simulink model "gm_uz_pmsm_model_vnl"  (R2023b)
settings: Solver=FixedStepAuto  StartTime=0.0  StopTime=0.05  RelTol=1e-3
PreLoadFcn:
  | uz_pmsm_model_init_parameter
PostLoadFcn:
  | % Import the data from Excel for a lookup table
  | FluxMapData = readtable('C:\Users\Philipp\ultrazohm\ultrazohm_sw\ip_cores\uz_pmsm_model\FluxMapData_2023-05-26_13-07-57.csv');
  | % Row indices for lookup table
  | d_current_in_d_axis = FluxMapData(8:27,1:end);
  | % Column indices for lookup table
  | q_current_in_d_axis = FluxMapData(29:48,1:end);
  | % Output values for lookup table
  | d_Flux_d_axis = FluxMapData(50:69,1:end);
undefined symbols (not defined in the file or in its folder): ad1, ad2, ad3, ad4, ad5, ad6, aq1, aq2, aq3, aq4, aq5, aq6, d_current_d_Flux, d_current_q_Flux, entkopplung_dynamic, entkopplung_linear, entkopplung_static, Fid1_Giq1, Fid2_Giq2, Flux_d, Flux_q, friction_coefficient, inertia, Ki_Bo_d, Ki_Bo_q, Kp_Bo_d, Kp_Bo_q, L_d, L_q, Ldq, parameter_nachfuerung, polepair, praediktion_entkopplung_nonlinear, psi_pm, q_current_d_Flux, q_current_q_Flux, R_1, simulate_mechanical, simulate_nonlinear_modell, simulate_open_loop, static_friction_torque, tau_sum, ts, ts_regler
libraries: hdlmdlgenlib x16, slpidlib x6, simulink x4
(part 4 of 5)

== system gm_uz_pmsm_model_vnl/uz_pmsm_model/Product9 ==
  In1 : Inport
  In2 : Inport  Port=2
  Product9 : Product  Inputs=**  OutDataTypeStr=single  SampleTime=1e-08
  Product9_pd1 : Delay  DelayLength=6
  Out1 : Outport
  wires:
  Product9_pd1/1 -> Out1/1
  Product9/1 -> Product9_pd1/1
  In2/1 -> Product9/2
  In1/1 -> Product9/1

== system gm_uz_pmsm_model_vnl/uz_pmsm_model/Product91 ==
  In1 : Inport
  In2 : Inport  Port=2
  Product91 : Product  Inputs=**  OutDataTypeStr=single  SampleTime=1e-08
  Product91_pd1 : Delay  DelayLength=6
  Out1 : Outport
  wires:
  Product91_pd1/1 -> Out1/1
  Product91/1 -> Product91_pd1/1
  In2/1 -> Product91/2
  In1/1 -> Product91/1

== system gm_uz_pmsm_model_vnl/uz_pmsm_model/Product92 ==
  In1 : Inport
  In2 : Inport  Port=2
  Product92 : Product  Inputs=**  OutDataTypeStr=single  SampleTime=1e-08
  Product92_pd1 : Delay  DelayLength=6
  Out1 : Outport
  wires:
  Product92_pd1/1 -> Out1/1
  Product92/1 -> Product92_pd1/1
  In2/1 -> Product92/2
  In1/1 -> Product92/1

== system gm_uz_pmsm_model_vnl/uz_pmsm_model/Reciprocal1_recip ==
  In1 : Inport
  Reciprocal1_recip : Math  Operator=reciprocal  SampleTime=1e-08
  Reciprocal1_recip_pd1 : Delay  DelayLength=16
  Out1 : Outport
  wires:
  Reciprocal1_recip_pd1/1 -> Out1/1
  Reciprocal1_recip/1 -> Reciprocal1_recip_pd1/1
  In1/1 -> Reciprocal1_recip/1

== system gm_uz_pmsm_model_vnl/uz_pmsm_model/Reciprocal1_recip1 ==
  In1 : Inport
  Reciprocal1_recip1 : Math  Operator=reciprocal  SampleTime=1e-08
  Reciprocal1_recip1_pd1 : Delay  DelayLength=16
  Out1 : Outport
  wires:
  Reciprocal1_recip1_pd1/1 -> Out1/1
  Reciprocal1_recip1/1 -> Reciprocal1_recip1_pd1/1
  In1/1 -> Reciprocal1_recip1/1

== system gm_uz_pmsm_model_vnl/uz_pmsm_model/Reciprocal_recip ==
  In1 : Inport
  Reciprocal_recip : Math  Operator=reciprocal  SampleTime=1e-08
  Reciprocal_recip_pd1 : Delay  DelayLength=16
  Out1 : Outport
  wires:
  Reciprocal_recip_pd1/1 -> Out1/1
  Reciprocal_recip/1 -> Reciprocal_recip_pd1/1
  In1/1 -> Reciprocal_recip/1

== system gm_uz_pmsm_model_vnl/uz_pmsm_model/Reciprocal_recip1 ==
  In1 : Inport
  Reciprocal_recip1 : Math  Operator=reciprocal  SampleTime=1e-08
  Reciprocal_recip1_pd1 : Delay  DelayLength=16
  Out1 : Outport
  wires:
  Reciprocal_recip1_pd1/1 -> Out1/1
  Reciprocal_recip1/1 -> Reciprocal_recip1_pd1/1
  In1/1 -> Reciprocal_recip1/1

== system gm_uz_pmsm_model_vnl/uz_pmsm_model/Sign1 ==
  In1 : Inport
  Sign1 : Signum  SampleTime=1e-08
  Out1 : Outport
  wires:
  Sign1/1 -> Out1/1
  In1/1 -> Sign1/1

== system gm_uz_pmsm_model_vnl/uz_pmsm_model/Sum ==
  In1 : Inport
  In2 : Inport  Port=2
  Sum : Sum  OutDataTypeStr=single  SampleTime=1e-08
  Sum_pd1 : Delay  DelayLength=6
  Out1 : Outport
  wires:
  Sum_pd1/1 -> Out1/1
  Sum/1 -> Sum_pd1/1
  In2/1 -> Sum/2
  In1/1 -> Sum/1

== system gm_uz_pmsm_model_vnl/uz_pmsm_model/Sum1 ==
  In1 : Inport
  In2 : Inport  Port=2
  Sum1 : Sum  Inputs=+-  OutDataTypeStr=single  SampleTime=1e-08
  Sum1_pd1 : Delay  DelayLength=6
  Out1 : Outport
  wires:
  Sum1_pd1/1 -> Out1/1
  Sum1/1 -> Sum1_pd1/1
  In2/1 -> Sum1/2
  In1/1 -> Sum1/1

== system gm_uz_pmsm_model_vnl/uz_pmsm_model/Sum10 ==
  In1 : Inport
  In2 : Inport  Port=2
  Sum10 : Sum  Inputs=+-  OutDataTypeStr=single  SampleTime=1e-08
  Sum10_pd1 : Delay  DelayLength=6
  Out1 : Outport
  wires:
  Sum10_pd1/1 -> Out1/1
  Sum10/1 -> Sum10_pd1/1
  In2/1 -> Sum10/2
  In1/1 -> Sum10/1

== system gm_uz_pmsm_model_vnl/uz_pmsm_model/Sum101 ==
  In1 : Inport
  In2 : Inport  Port=2
  Sum101 : Sum  Inputs=+-  OutDataTypeStr=single  SampleTime=1e-08
  Sum101_pd1 : Delay  DelayLength=6
  Out1 : Outport
  wires:
  Sum101_pd1/1 -> Out1/1
  Sum101/1 -> Sum101_pd1/1
  In2/1 -> Sum101/2
  In1/1 -> Sum101/1

== system gm_uz_pmsm_model_vnl/uz_pmsm_model/Sum11 ==
  In1 : Inport
  In2 : Inport  Port=2
  Sum11 : Sum  Inputs=+-  OutDataTypeStr=single  SampleTime=1e-08
  Sum11_pd1 : Delay  DelayLength=6
  Out1 : Outport
  wires:
  Sum11_pd1/1 -> Out1/1
  Sum11/1 -> Sum11_pd1/1
  In2/1 -> Sum11/2
  In1/1 -> Sum11/1

== system gm_uz_pmsm_model_vnl/uz_pmsm_model/Sum12 ==
  In1 : Inport
  In2 : Inport  Port=2
  Sum12 : Sum  OutDataTypeStr=single  SampleTime=1e-08
  Sum12_pd1 : Delay  DelayLength=6
  Out1 : Outport
  wires:
  Sum12_pd1/1 -> Out1/1
  Sum12/1 -> Sum12_pd1/1
  In2/1 -> Sum12/2
  In1/1 -> Sum12/1

== system gm_uz_pmsm_model_vnl/uz_pmsm_model/Sum13 ==
  In1 : Inport
  In2 : Inport  Port=2
  Sum13 : Sum  OutDataTypeStr=single  SampleTime=1e-08
  Sum13_pd1 : Delay  DelayLength=6
  Out1 : Outport
  wires:
  Sum13_pd1/1 -> Out1/1
  Sum13/1 -> Sum13_pd1/1
  In2/1 -> Sum13/2
  In1/1 -> Sum13/1

== system gm_uz_pmsm_model_vnl/uz_pmsm_model/Sum14 ==
  In1 : Inport
  In2 : Inport  Port=2
  Sum14 : Sum  Inputs=+-  OutDataTypeStr=single  SampleTime=1e-08
  Sum14_pd1 : Delay  DelayLength=6
  Out1 : Outport
  wires:
  Sum14_pd1/1 -> Out1/1
  Sum14/1 -> Sum14_pd1/1
  In2/1 -> Sum14/2
  In1/1 -> Sum14/1

== system gm_uz_pmsm_model_vnl/uz_pmsm_model/Sum2 ==
  In1 : Inport
  In2 : Inport  Port=2
  Sum2 : Sum  Inputs=+-  OutDataTypeStr=single  SampleTime=1e-08
  Sum2_pd1 : Delay  DelayLength=6
  Out1 : Outport
  wires:
  Sum2_pd1/1 -> Out1/1
  Sum2/1 -> Sum2_pd1/1
  In2/1 -> Sum2/2
  In1/1 -> Sum2/1

== system gm_uz_pmsm_model_vnl/uz_pmsm_model/Sum21 ==
  In1 : Inport
  In2 : Inport  Port=2
  Sum21 : Sum  Inputs=+-  OutDataTypeStr=single  SampleTime=1e-08
  Sum21_pd1 : Delay  DelayLength=6
  Out1 : Outport
  wires:
  Sum21_pd1/1 -> Out1/1
  Sum21/1 -> Sum21_pd1/1
  In2/1 -> Sum21/2
  In1/1 -> Sum21/1

== system gm_uz_pmsm_model_vnl/uz_pmsm_model/Sum22 ==
  In1 : Inport
  In2 : Inport  Port=2
  Sum22 : Sum  Inputs=+-  OutDataTypeStr=single  SampleTime=1e-08
  Sum22_pd1 : Delay  DelayLength=6
  Out1 : Outport
  wires:
  Sum22_pd1/1 -> Out1/1
  Sum22/1 -> Sum22_pd1/1
  In2/1 -> Sum22/2
  In1/1 -> Sum22/1

== system gm_uz_pmsm_model_vnl/uz_pmsm_model/Sum23 ==
  In1 : Inport
  In2 : Inport  Port=2
  Sum23 : Sum  Inputs=+-  OutDataTypeStr=single  SampleTime=1e-08
  Sum23_pd1 : Delay  DelayLength=6
  Out1 : Outport
  wires:
  Sum23_pd1/1 -> Out1/1
  Sum23/1 -> Sum23_pd1/1
  In2/1 -> Sum23/2
  In1/1 -> Sum23/1

== system gm_uz_pmsm_model_vnl/uz_pmsm_model/Sum24 ==
  In1 : Inport
  In2 : Inport  Port=2
  Sum24 : Sum  Inputs=+-  OutDataTypeStr=single  SampleTime=1e-08
  Sum24_pd1 : Delay  DelayLength=6
  Out1 : Outport
  wires:
  Sum24_pd1/1 -> Out1/1
  Sum24/1 -> Sum24_pd1/1
  In2/1 -> Sum24/2
  In1/1 -> Sum24/1

== system gm_uz_pmsm_model_vnl/uz_pmsm_model/Sum3 ==
  In1 : Inport
  In2 : Inport  Port=2
  Sum3 : Sum  Inputs=+-  OutDataTypeStr=single  SampleTime=1e-08
  Sum3_pd1 : Delay  DelayLength=6
  Out1 : Outport
  wires:
  Sum3_pd1/1 -> Out1/1
  Sum3/1 -> Sum3_pd1/1
  In2/1 -> Sum3/2
  In1/1 -> Sum3/1

== system gm_uz_pmsm_model_vnl/uz_pmsm_model/Sum31 ==
  In1 : Inport
  In2 : Inport  Port=2
  Sum31 : Sum  Inputs=+-  OutDataTypeStr=single  SampleTime=1e-08
  Sum31_pd1 : Delay  DelayLength=6
  Out1 : Outport
  wires:
  Sum31_pd1/1 -> Out1/1
  Sum31/1 -> Sum31_pd1/1
  In2/1 -> Sum31/2
  In1/1 -> Sum31/1

== system gm_uz_pmsm_model_vnl/uz_pmsm_model/Sum32 ==
  In1 : Inport
  In2 : Inport  Port=2
  Sum32 : Sum  OutDataTypeStr=single  SampleTime=1e-08
  Sum32_pd1 : Delay  DelayLength=6
  Out1 : Outport
  wires:
  Sum32_pd1/1 -> Out1/1
  Sum32/1 -> Sum32_pd1/1
  In2/1 -> Sum32/2
  In1/1 -> Sum32/1

== system gm_uz_pmsm_model_vnl/uz_pmsm_model/Sum33 ==
  In1 : Inport
  In2 : Inport  Port=2
  Sum33 : Sum  Inputs=+-  OutDataTypeStr=single  SampleTime=1e-08
  Sum33_pd1 : Delay  DelayLength=6
  Out1 : Outport
  wires:
  Sum33_pd1/1 -> Out1/1
  Sum33/1 -> Sum33_pd1/1
  In2/1 -> Sum33/2
  In1/1 -> Sum33/1

== system gm_uz_pmsm_model_vnl/uz_pmsm_model/Sum3_stage2 ==
  In1 : Inport
  In2 : Inport  Port=2
  Sum3_stage2 : Sum  OutDataTypeStr=single  SampleTime=1e-08
  Sum3_stage2_pd1 : Delay  DelayLength=6
  Out1 : Outport
  wires:
  Sum3_stage2_pd1/1 -> Out1/1
  Sum3_stage2/1 -> Sum3_stage2_pd1/1
  In2/1 -> Sum3_stage2/2
  In1/1 -> Sum3_stage2/1

== system gm_uz_pmsm_model_vnl/uz_pmsm_model/Sum3_stage21 ==
  In1 : Inport
  In2 : Inport  Port=2
  Sum3_stage21 : Sum  Inputs=+-  OutDataTypeStr=single  SampleTime=1e-08
  Sum3_stage21_pd1 : Delay  DelayLength=6
  Out1 : Outport
  wires:
  Sum3_stage21_pd1/1 -> Out1/1
  Sum3_stage21/1 -> Sum3_stage21_pd1/1
  In2/1 -> Sum3_stage21/2
  In1/1 -> Sum3_stage21/1

== system gm_uz_pmsm_model_vnl/uz_pmsm_model/Sum3_stage3 ==
  In1 : Inport
  In2 : Inport  Port=2
  Sum3_stage3 : Sum  Inputs=+-  OutDataTypeStr=single  SampleTime=1e-08
  Sum3_stage3_pd1 : Delay  DelayLength=6
  Out1 : Outport
  wires:
  Sum3_stage3_pd1/1 -> Out1/1
  Sum3_stage3/1 -> Sum3_stage3_pd1/1
  In2/1 -> Sum3_stage3/2
  In1/1 -> Sum3_stage3/1

== system gm_uz_pmsm_model_vnl/uz_pmsm_model/Sum3_stage31 ==
  In1 : Inport
  In2 : Inport  Port=2
  Sum3_stage31 : Sum  OutDataTypeStr=single  SampleTime=1e-08
  Sum3_stage31_pd1 : Delay  DelayLength=6
  Out1 : Outport
  wires:
  Sum3_stage31_pd1/1 -> Out1/1
  Sum3_stage31/1 -> Sum3_stage31_pd1/1
  In2/1 -> Sum3_stage31/2
  In1/1 -> Sum3_stage31/1

== system gm_uz_pmsm_model_vnl/uz_pmsm_model/Sum4 ==
  In1 : Inport
  In2 : Inport  Port=2
  Sum4 : Sum  OutDataTypeStr=single  SampleTime=1e-08
  Sum4_pd1 : Delay  DelayLength=6
  Out1 : Outport
  wires:
  Sum4_pd1/1 -> Out1/1
  Sum4/1 -> Sum4_pd1/1
  In2/1 -> Sum4/2
  In1/1 -> Sum4/1

== system gm_uz_pmsm_model_vnl/uz_pmsm_model/Sum41 ==
  In1 : Inport
  In2 : Inport  Port=2
  Sum41 : Sum  OutDataTypeStr=single  SampleTime=1e-08
  Sum41_pd1 : Delay  DelayLength=6
  Out1 : Outport
  wires:
  Sum41_pd1/1 -> Out1/1
  Sum41/1 -> Sum41_pd1/1
  In2/1 -> Sum41/2
  In1/1 -> Sum41/1

== system gm_uz_pmsm_model_vnl/uz_pmsm_model/Sum4_stage2 ==
  In1 : Inport
  In2 : Inport  Port=2
  Sum4_stage2 : Sum  Inputs=+-  OutDataTypeStr=single  SampleTime=1e-08
  Sum4_stage2_pd1 : Delay  DelayLength=6
  Out1 : Outport
  wires:
  Sum4_stage2_pd1/1 -> Out1/1
  Sum4_stage2/1 -> Sum4_stage2_pd1/1
  In2/1 -> Sum4_stage2/2
  In1/1 -> Sum4_stage2/1

== system gm_uz_pmsm_model_vnl/uz_pmsm_model/Sum4_stage3 ==
  In1 : Inport
  In2 : Inport  Port=2
  Sum4_stage3 : Sum  Inputs=+-  OutDataTypeStr=single  SampleTime=1e-08
  Sum4_stage3_pd1 : Delay  DelayLength=6
  Out1 : Outport
  wires:
  Sum4_stage3_pd1/1 -> Out1/1
  Sum4_stage3/1 -> Sum4_stage3_pd1/1
  In2/1 -> Sum4_stage3/2
  In1/1 -> Sum4_stage3/1

== system gm_uz_pmsm_model_vnl/uz_pmsm_model/Sum5 ==
  In1 : Inport
  In2 : Inport  Port=2
  Sum5 : Sum  OutDataTypeStr=single  SampleTime=1e-08
  Sum5_pd1 : Delay  DelayLength=6
  Out1 : Outport
  wires:
  Sum5_pd1/1 -> Out1/1
  Sum5/1 -> Sum5_pd1/1
  In2/1 -> Sum5/2
  In1/1 -> Sum5/1

== system gm_uz_pmsm_model_vnl/uz_pmsm_model/Sum51 ==
  In1 : Inport
  In2 : Inport  Port=2
  Sum51 : Sum  Inputs=+-  OutDataTypeStr=single  SampleTime=1e-08
  Sum51_pd1 : Delay  DelayLength=6
  Out1 : Outport
  wires:
  Sum51_pd1/1 -> Out1/1
  Sum51/1 -> Sum51_pd1/1
  In2/1 -> Sum51/2
  In1/1 -> Sum51/1

== system gm_uz_pmsm_model_vnl/uz_pmsm_model/Sum52 ==
  In1 : Inport
  In2 : Inport  Port=2
  Sum52 : Sum  OutDataTypeStr=single  SampleTime=1e-08
  Sum52_pd1 : Delay  DelayLength=6
  Out1 : Outport
  wires:
  Sum52_pd1/1 -> Out1/1
  Sum52/1 -> Sum52_pd1/1
  In2/1 -> Sum52/2
  In1/1 -> Sum52/1

== system gm_uz_pmsm_model_vnl/uz_pmsm_model/Sum53 ==
  In1 : Inport
  In2 : Inport  Port=2
  Sum53 : Sum  OutDataTypeStr=single  SampleTime=1e-08
  Sum53_pd1 : Delay  DelayLength=6
  Out1 : Outport
  wires:
  Sum53_pd1/1 -> Out1/1
  Sum53/1 -> Sum53_pd1/1
  In2/1 -> Sum53/2
  In1/1 -> Sum53/1

== system gm_uz_pmsm_model_vnl/uz_pmsm_model/Sum6 ==
  In1 : Inport
  In2 : Inport  Port=2
  Sum6 : Sum  Inputs=+-  OutDataTypeStr=single  SampleTime=1e-08
  Sum6_pd1 : Delay  DelayLength=6
  Out1 : Outport
  wires:
  Sum6_pd1/1 -> Out1/1
  Sum6/1 -> Sum6_pd1/1
  In2/1 -> Sum6/2
  In1/1 -> Sum6/1

== system gm_uz_pmsm_model_vnl/uz_pmsm_model/Sum7 ==
  In1 : Inport
  In2 : Inport  Port=2
  Sum7 : Sum  Inputs=+-  OutDataTypeStr=single  SampleTime=1e-08
  Sum7_pd1 : Delay  DelayLength=6
  Out1 : Outport
  wires:
  Sum7_pd1/1 -> Out1/1
  Sum7/1 -> Sum7_pd1/1
  In2/1 -> Sum7/2
  In1/1 -> Sum7/1

== system gm_uz_pmsm_model_vnl/uz_pmsm_model/Sum71 ==
  In1 : Inport
  In2 : Inport  Port=2
  Sum71 : Sum  Inputs=+-  OutDataTypeStr=single  SampleTime=1e-08
  Sum71_pd1 : Delay  DelayLength=6
  Out1 : Outport
  wires:
  Sum71_pd1/1 -> Out1/1
  Sum71/1 -> Sum71_pd1/1
  In2/1 -> Sum71/2
  In1/1 -> Sum71/1

== system gm_uz_pmsm_model_vnl/uz_pmsm_model/Sum8 ==
  In1 : Inport
  In2 : Inport  Port=2
  Sum8 : Sum  Inputs=+-  OutDataTypeStr=single  SampleTime=1e-08
  Sum8_pd1 : Delay  DelayLength=6
  Out1 : Outport
  wires:
  Sum8_pd1/1 -> Out1/1
  Sum8/1 -> Sum8_pd1/1
  In2/1 -> Sum8/2
  In1/1 -> Sum8/1

== system gm_uz_pmsm_model_vnl/uz_pmsm_model/Tanh ==
  In1 : Inport
  Tanh : Trigonometry  Operator=tanh  SampleTime=1e-08
  Tanh_pd1 : Delay  DelayLength=25
  Out1 : Outport
  wires:
  Tanh_pd1/1 -> Out1/1
  Tanh/1 -> Tanh_pd1/1
  In1/1 -> Tanh/1

== system gm_uz_pmsm_model_vnl/uz_pmsm_model/Tanh1 ==
  In1 : Inport
  Tanh1 : Trigonometry  Operator=tanh  SampleTime=1e-08
  Tanh1_pd1 : Delay  DelayLength=25
  Out1 : Outport
  wires:
  Tanh1_pd1/1 -> Out1/1
  Tanh1/1 -> Tanh1_pd1/1
  In1/1 -> Tanh1/1

== system gm_uz_pmsm_model_vnl/uz_pmsm_model/Tanh11 ==
  In1 : Inport
  Tanh11 : Trigonometry  Operator=cosh  SampleTime=1e-08
  Tanh11_pd1 : Delay  DelayLength=17
  Out1 : Outport
  wires:
  Tanh11_pd1/1 -> Out1/1
  Tanh11/1 -> Tanh11_pd1/1
  In1/1 -> Tanh11/1

== system gm_uz_pmsm_model_vnl/uz_pmsm_model/Tanh12 ==
  In1 : Inport
  Tanh12 : Trigonometry  Operator=tanh  SampleTime=1e-08
  Tanh12_pd1 : Delay  DelayLength=25
  Out1 : Outport
  wires:
  Tanh12_pd1/1 -> Out1/1
  Tanh12/1 -> Tanh12_pd1/1
  In1/1 -> Tanh12/1

== system gm_uz_pmsm_model_vnl/uz_pmsm_model/Tanh13 ==
  In1 : Inport
  Tanh13 : Trigonometry  Operator=cosh  SampleTime=1e-08
  Tanh13_pd1 : Delay  DelayLength=17
  Out1 : Outport
  wires:
  Tanh13_pd1/1 -> Out1/1
  Tanh13/1 -> Tanh13_pd1/1
  In1/1 -> Tanh13/1

== system gm_uz_pmsm_model_vnl/uz_pmsm_model/Tanh2 ==
  In1 : Inport
  Tanh2 : Trigonometry  Operator=cosh  SampleTime=1e-08
  Tanh2_pd1 : Delay  DelayLength=17
  Out1 : Outport
  wires:
  Tanh2_pd1/1 -> Out1/1
  Tanh2/1 -> Tanh2_pd1/1
  In1/1 -> Tanh2/1

== system gm_uz_pmsm_model_vnl/uz_pmsm_model/Tanh21 ==
  In1 : Inport
  Tanh21 : Trigonometry  Operator=cosh  SampleTime=1e-08
  Tanh21_pd1 : Delay  DelayLength=17
  Out1 : Outport
  wires:
  Tanh21_pd1/1 -> Out1/1
  Tanh21/1 -> Tanh21_pd1/1
  In1/1 -> Tanh21/1

== system gm_uz_pmsm_model_vnl/uz_pmsm_model/Tanh3 ==
  In1 : Inport
  Tanh3 : Trigonometry  Operator=cosh  SampleTime=1e-08
  Tanh3_pd1 : Delay  DelayLength=17
  Out1 : Outport
  wires:
  Tanh3_pd1/1 -> Out1/1
  Tanh3/1 -> Tanh3_pd1/1
  In1/1 -> Tanh3/1

== system gm_uz_pmsm_model_vnl/uz_pmsm_model/Tanh31 ==
  In1 : Inport
  Tanh31 : Trigonometry  Operator=cosh  SampleTime=1e-08
  Tanh31_pd1 : Delay  DelayLength=17
  Out1 : Outport
  wires:
  Tanh31_pd1/1 -> Out1/1
  Tanh31/1 -> Tanh31_pd1/1
  In1/1 -> Tanh31/1

== system gm_uz_pmsm_model_vnl/uz_pmsm_model/Tanh4 ==
  In1 : Inport
  Tanh4 : Trigonometry  Operator=cosh  SampleTime=1e-08
  Tanh4_pd1 : Delay  DelayLength=17
  Out1 : Outport
  wires:
  Tanh4_pd1/1 -> Out1/1
  Tanh4/1 -> Tanh4_pd1/1
  In1/1 -> Tanh4/1

== system gm_uz_pmsm_model_vnl/uz_pmsm_model/Tanh41 ==
  In1 : Inport
  Tanh41 : Trigonometry  Operator=cosh  SampleTime=1e-08
  Tanh41_pd1 : Delay  DelayLength=17
  Out1 : Outport
  wires:
  Tanh41_pd1/1 -> Out1/1
  Tanh41/1 -> Tanh41_pd1/1
  In1/1 -> Tanh41/1

== system gm_uz_pmsm_model_vnl/uz_pmsm_model/Tanh5 ==
  In1 : Inport
  Tanh5 : Trigonometry  Operator=tanh  SampleTime=1e-08
  Tanh5_pd1 : Delay  DelayLength=25
  Out1 : Outport
  wires:
  Tanh5_pd1/1 -> Out1/1
  Tanh5/1 -> Tanh5_pd1/1
  In1/1 -> Tanh5/1

== system gm_uz_pmsm_model_vnl/uz_pmsm_model/abs ==
  In1 : Inport
  abs : Abs  SampleTime=1e-08  OutDataTypeStr=single  SaturateOnIntegerOverflow=off
  Out1 : Outport
  wires:
  abs/1 -> Out1/1
  In1/1 -> abs/1

== system gm_uz_pmsm_model_vnl/uz_pmsm_model/abs1 ==
  In1 : Inport
  abs1 : Abs  SampleTime=1e-08  OutDataTypeStr=single  SaturateOnIntegerOverflow=off
  Out1 : Outport
  wires:
  abs1/1 -> Out1/1
  In1/1 -> abs1/1

== system gm_uz_pmsm_model_vnl/uz_pmsm_model/abs2 ==
  In1 : Inport
  abs2 : Abs  SampleTime=1e-08  OutDataTypeStr=single  SaturateOnIntegerOverflow=off
  Out1 : Outport
  wires:
  abs2/1 -> Out1/1
  In1/1 -> abs2/1

== system gm_uz_pmsm_model_vnl/uz_pmsm_model/abs3 ==
  In1 : Inport
  abs3 : Abs  SampleTime=1e-08  OutDataTypeStr=single  SaturateOnIntegerOverflow=off
  Out1 : Outport
  wires:
  abs3/1 -> Out1/1
  In1/1 -> abs3/1

== system gm_uz_pmsm_model_vnl/uz_pmsm_model/abs4 ==
  In1 : Inport
  abs4 : Abs  SampleTime=1e-08  OutDataTypeStr=single  SaturateOnIntegerOverflow=off
  Out1 : Outport
  wires:
  abs4/1 -> Out1/1
  In1/1 -> abs4/1

== system gm_uz_pmsm_model_vnl/uz_pmsm_model/abs5 ==
  In1 : Inport
  abs5 : Abs  SampleTime=1e-08  OutDataTypeStr=single  SaturateOnIntegerOverflow=off
  Out1 : Outport
  wires:
  abs5/1 -> Out1/1
  In1/1 -> abs5/1

== system gm_uz_pmsm_model_vnl/uz_pmsm_model/abs6 ==
  In1 : Inport
  abs6 : Abs  SampleTime=1e-08  OutDataTypeStr=single  SaturateOnIntegerOverflow=off
  Out1 : Outport
  wires:
  abs6/1 -> Out1/1
  In1/1 -> abs6/1

== system gm_uz_pmsm_model_vnl/uz_pmsm_model/abs7 ==
  In1 : Inport
  abs7 : Abs  SampleTime=1e-08  OutDataTypeStr=single  SaturateOnIntegerOverflow=off
  Out1 : Outport
  wires:
  abs7/1 -> Out1/1
  In1/1 -> abs7/1

== system gm_uz_pmsm_model_vnl/uz_pmsm_model/abs8 ==
  In1 : Inport
  abs8 : Abs  SampleTime=1e-08  OutDataTypeStr=single  SaturateOnIntegerOverflow=off
  Out1 : Outport
  wires:
  abs8/1 -> Out1/1
  In1/1 -> abs8/1

== system gm_uz_pmsm_model_vnl/uz_pmsm_model/abs9 ==
  In1 : Inport
  abs9 : Abs  SampleTime=1e-08  OutDataTypeStr=single  SaturateOnIntegerOverflow=off
  Out1 : Outport
  wires:
  abs9/1 -> Out1/1
  In1/1 -> abs9/1

== system gm_uz_pmsm_model_vnl/uz_pmsm_model_vnl/mechanical_system ==
  note: This delay breaks the algebraic loop between mechanical and electrical system.
      | Introduces a delay of 500ns.
  reset : Inport
  M_Mi : Inport  Port=2
  mu : Inport  Port=3
  M_n0 : Inport  Port=4
  reciprocal_J : Inport  Port=5
  load_torque : Inport  Port=6
  Abs : Abs  SaturateOnIntegerOverflow=off
  Delay : Delay  DelayLength=1
  Product11 : Product
  Product12 : Product
  Product4 : Product
  Sign1 : Signum
  Sum : Sum  Inputs=|+-
  Sum1 : Sum  Inputs=|+-
  Sum5 : Sum  Inputs=|++
  integrator1 : Subsystem
  omega_mech : Outport
  wires:
  Delay/1 -> Sum1/1
  Product4/1 -> Sum/2
  Sum/1 -> Delay/1
  load_torque/1 -> Sum1/2
  Sum1/1 -> Product11/2
  M_Mi/1 -> Sum/1
  reciprocal_J/1 -> Product11/1
  M_n0/1 -> Sum5/2
  mu/1 -> Product12/1
  Product12/1 -> Sum5/1
  reset/1 -> integrator1/1(reset)
  Abs/1 -> Product12/2
  integrator1/1(outt) -> omega_mech/1, Abs/1, Sign1/1
  Sign1/1 -> Product4/2
  Sum5/1 -> Product4/1
  Product11/1 -> integrator1/2(in)

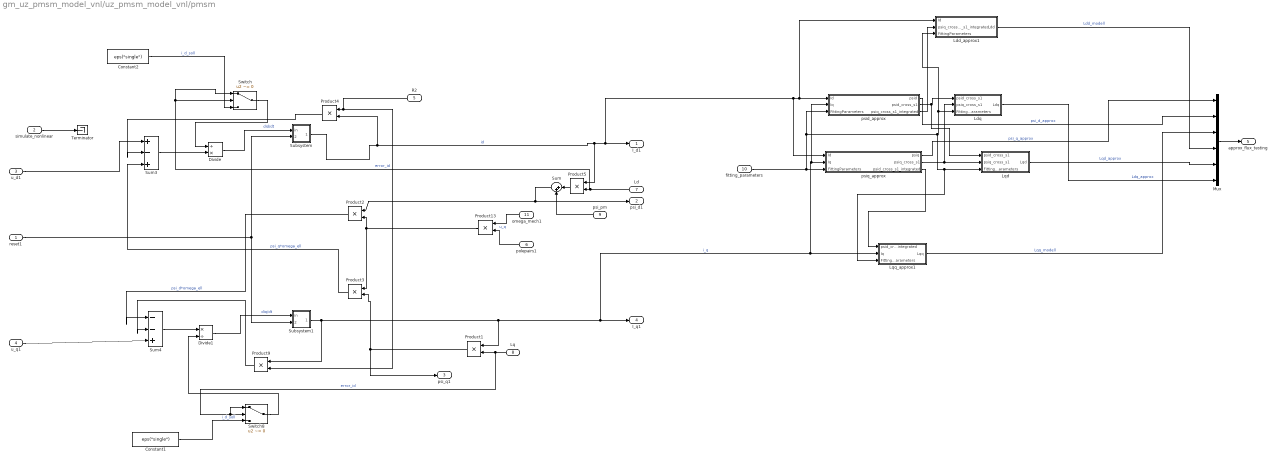
== system gm_uz_pmsm_model_vnl/uz_pmsm_model_vnl/pmsm ==
  reset1 : Inport
  simulate_nonlinear : Inport  Port=2
  u_d1 : Inport  Port=3
  u_q1 : Inport  Port=4
  R2 : Inport  Port=5
  polepairs1 : Inport  Port=6
  Ld : Inport  Port=7
  Lq : Inport  Port=8
  psi_pm : Inport  Port=9
  fitting_parameters : Inport  Port=10
  omega_mech1 : Inport  Port=11
  Constant1 : Constant  Value="eps(\"single\")"  OutDataTypeStr=single  SampleTime=ts
  Constant2 : Constant  Value="eps(\"single\")"  OutDataTypeStr=single  SampleTime=ts
  Divide : Product  Inputs=/*  OutDataTypeStr=Inherit: Same as first input
  Divide1 : Product  Inputs=*/  OutDataTypeStr=Inherit: Same as first input
  Ldd_approx1 : Subsystem
  Ldq : Subsystem
  Lqd : Subsystem
  Lqq_approx1 : Subsystem
  Mux : Mux  Inputs=6
  Product1 : Product
  Product{2,4..5,9,13} (5 alike) : Product  OutDataTypeStr=Inherit: Same as first input
  Product3 : Product
  Subsystem : Subsystem
  Subsystem1 : Subsystem
  Sum : Sum  Inputs=|++  OutDataTypeStr=Inherit: Same as first input
  Sum3 : Sum  Inputs=|+-+  OutDataTypeStr=Inherit: Same as first input
  Sum4 : Sum  Inputs=|--+
  Switch : Switch  Criteria=u2 ~= 0  Threshold="eps(\"single\")"  SaturateOnIntegerOverflow=off  InputSameDT=off
  Switch8 : Switch  Criteria=u2 ~= 0  SaturateOnIntegerOverflow=off  InputSameDT=off
  Terminator : Terminator
  psid_approx : Subsystem
  psiq_approx : Subsystem
  I_d1 : Outport
  psi_d1 : Outport  Port=2
  psi_q1 : Outport  Port=3
  I_q1 : Outport  Port=4
  approx_flux_testing : Outport  Port=5
  wires:
  fitting_parameters/1 -> psiq_approx/3(FittingParameters), psid_approx/3(FittingParameters), Ldq/3(FittingParameters), Ldd_approx1/3(FittingParameters), Lqd/3(FittingParameters), Lqq_approx1/3(FittingParameters)
  Mux/1 -> approx_flux_testing/1
  Ldd_approx1/1(Ldd) -> Mux/4  "Ldd_modell"
  psiq_approx/3(psid_cross_s1_integrated) -> Lqq_approx1/1(psid_cross_s1_integrated)
  psid_approx/3(psiq_cross_s1_integrated) -> Ldd_approx1/2(psiq_cross_s1_integrated)
  simulate_nonlinear/1 -> Terminator/1
  Ldq/1(Ldq) -> Mux/6  "Ldq_approx"
  Lqd/1(Lqd) -> Mux/5  "Lqd_approx"
  psid_approx/1(psid) -> Mux/2  "psi_d_approx"
  psiq_approx/1(psiq) -> Mux/1  "psi_q_approx"
  psiq_approx/2(psiq_cross_s1) -> Ldq/2(psiq_cross_s1), Lqd/2(psiq_cross_s1)
  psid_approx/2(psid_cross_s1) -> Ldq/1(psid_cross_s1), Lqd/1(psid_cross_s1)
  Constant2/1 -> Switch/3  "i_d_soll"
  Constant1/1 -> Switch8/3  "i_d_soll"
  Switch/1 -> Divide/1
  Ld/1 -> Product5/2, Switch/1, Switch/2  "error_id"
  Switch8/1 -> Divide1/2
  Lq/1 -> Product1/2, Switch8/2, Switch8/1  "error_id"
  Product1/1 -> psi_q1/1, Product3/2
  psi_pm/1 -> Sum/2
  Product5/1 -> Sum/1
  Sum/1 -> psi_d1/1, Product2/1
  Lqq_approx1/1(Lqq) -> Mux/3  "Lqq_modell"
  omega_mech1/1 -> Product13/1  "u_q"
  Product2/1 -> Sum4/1  "psi_d*omega_ell"
  Product4/1 -> Sum3/2
  Product3/1 -> Sum3/3  "psi_q*omega_ell"
  Subsystem1/1(outt) -> Product9/1, Product1/1, I_q1/1, Lqq_approx1/2(Iq), psiq_approx/2(Iq), psid_approx/2(Iq)  "i_q"
  Subsystem/1(outt) -> I_d1/1, psid_approx/1(Id), Ldd_approx1/1(Id), psiq_approx/1(Id), Product5/1, Product4/2  "id"
  R2/1 -> Product4/1, Product9/2
  u_d1/1 -> Sum3/1
  reset1/1 -> Subsystem1/2(reset), Subsystem/2(reset)
  Product9/1 -> Sum4/2
  Sum3/1 -> Divide/2
  Divide/1 -> Subsystem/1(in)  "did/dt"
  Product13/1 -> Product2/2, Product3/1
  polepairs1/1 -> Product13/2
  Divide1/1 -> Subsystem1/1(in)  "diq/dt"
  u_q1/1 -> Sum4/3
  Sum4/1 -> Divide1/1

== system gm_uz_pmsm_model_vnl/uz_pmsm_model_vnl/torque_calculation ==
  I_d : Inport
  psi_d : Inport  Port=2
  psi_q : Inport  Port=3
  polepairs : Inport  Port=4
  I_q : Inport  Port=5
  Factor : Gain  Gain=(3/2)
  Product2 : Product
  Product3 : Product
  Product9 : Product
  Sum3 : Sum  Inputs=-|+
  M_Mi : Outport
  wires:
  Factor/1 -> Product9/1  "M_Mi"
  polepairs/1 -> Product9/2
  Product9/1 -> M_Mi/1  "M_Mi"
  I_q/1 -> Product3/2
  I_d/1 -> Product2/1
  psi_d/1 -> Product3/1
  psi_q/1 -> Product2/2
  Product2/1 -> Sum3/1
  Product3/1 -> Sum3/2
  Sum3/1 -> Factor/1

== system gm_uz_pmsm_model_vnl/Compare/Assert_approx_flux_testing/RelErrCheck ==
  In1 : Inport
  In2 : Inport  Port=2
  "RelativeErrorCheck " : MATLAB Function  TreatAsAtomicUnit=on
  Out1 : Outport  VectorParamsAs1DForOutWhenUnconnected=off
  wires:
  "RelativeErrorCheck "/1(y) -> Out1/1
  In1/1 -> "RelativeErrorCheck "/1(P)
  In2/1 -> "RelativeErrorCheck "/2(R)

== system gm_uz_pmsm_model_vnl/Compare/Assert_outputs/RelErrCheck ==
  In1 : Inport
  In2 : Inport  Port=2
  "RelativeErrorCheck " : MATLAB Function  TreatAsAtomicUnit=on
  Out1 : Outport  VectorParamsAs1DForOutWhenUnconnected=off
  wires:
  "RelativeErrorCheck "/1(y) -> Out1/1
  In1/1 -> "RelativeErrorCheck "/1(P)
  In2/1 -> "RelativeErrorCheck "/2(R)

== system gm_uz_pmsm_model_vnl/Curren t_Controller_With_FluxMaps_OLD/Entkopplungen/Lineare_Entkopplung ==
  i_d : Inport
  i_q : Inport  Port=2
  omega_m : Inport  Port=3
  Constant1 : Constant  Value=psi_pm  SampleTime=-1
  Gain : Gain  Gain=L_q
  Gain1 : Gain  Gain=L_d
  Gain2 : Gain  Gain=polepair  OutDataTypeStr=Inherit: Same as input
  Product : Product
  Product1 : Product
  Sum6 : Sum  Inputs=|++
  u_d : Outport
  u_q : Outport  Port=2
  wires:
  omega_m/1 -> Gain2/1
  Sum6/1 -> Product1/1
  Product/1 -> u_d/1
  i_d/1 -> Gain1/1
  Constant1/1 -> Sum6/2
  i_q/1 -> Gain/1
  Product1/1 -> u_q/1
  Gain1/1 -> Sum6/1
  Gain2/1 -> Product1/2, Product/2
  Gain/1 -> Product/1

== system gm_uz_pmsm_model_vnl/Curren t_Controller_With_FluxMaps_OLD/Entkopplungen/decoupling_praediktion ==
  i_d : Inport
  u_d_1 : Inport  Port=2
  i_q : Inport  Port=3
  u_q_1 : Inport  Port=4
  omega_m : Inport  Port=5
  u_d_k : Inport  Port=6
  u_q_k : Inport  Port=7
  psi_q : Inport  Port=8
  psi_d : Inport  Port=9
  Gain : Gain  Gain=R_1
  Gain1 : Gain  Gain=R_1
  Gain2 : Gain  Gain=polepair
  Gain3 : Gain  Gain=ts_regler
  Gain4 : Gain  Gain=ts_regler
  Gain5 : Gain  Gain=ts_regler/2
  Gain6 : Gain  Gain=ts_regler/2
  Product{1..4} (4 alike) : Product
  Sum : Sum  Inputs=|+-
  Sum1 : Sum  Inputs=|+-
  Sum2 : Sum  Inputs=++|
  Sum3 : Sum  Inputs=|-+
  Sum4 : Sum  Inputs=++|
  Sum5 : Sum  Inputs=|++
  Sum6 : Sum  Inputs=++|
  Sum7 : Sum  Inputs=|++
  u_d_entk : Outport
  u_q_entk : Outport  Port=2
  wires:
  psi_q/1 -> Sum5/2, Product2/1
  psi_d/1 -> Product3/2, Sum4/1
  Gain2/1 -> Product1/2, Product4/1, Product3/1, Product2/2
  u_d_k/1 -> Sum/2
  Gain/1 -> Sum/1
  u_q_k/1 -> Sum1/1
  Gain1/1 -> Sum1/2
  Product3/1 -> Sum3/1
  Product2/1 -> Sum2/2
  Sum/1 -> Sum2/1
  Sum1/1 -> Sum3/2
  Sum3/1 -> Gain4/1
  Sum2/1 -> Gain3/1
  Gain3/1 -> Sum4/2
  Gain4/1 -> Sum5/1
  u_d_1/1 -> Gain5/1
  Sum4/1 -> Sum6/2
  u_q_1/1 -> Gain6/1
  Gain5/1 -> Sum6/1
  Sum5/1 -> Sum7/1
  Gain6/1 -> Sum7/2
  Sum6/1 -> Product1/1
  Sum7/1 -> Product4/2
  omega_m/1 -> Gain2/1
  i_d/1 -> Gain/1
  i_q/1 -> Gain1/1
  Product1/1 -> u_q_entk/1
  Product4/1 -> u_d_entk/1

== system gm_uz_pmsm_model_vnl/Curren t_Controller_With_FluxMaps_OLD/Entkopplungen/dynamic_nonlinear_entkopplung1 ==
  i_d : Inport
  i_q : Inport  Port=2
  psi_d : Inport  Port=3
  psi_q : Inport  Port=4
  Ldq_LUT : Inport  Port=5
  Lqd_LUT : Inport  Port=6
  omega_m : Inport  Port=7
  Gain2 : Gain  Gain=polepair
  Product{,1..3} (4 alike) : Product
  Sum1 : Sum  Inputs=++|
  Sum6 : Sum  Inputs=++|
  u_d : Outport
  u_q : Outport  Port=2
  wires:
  psi_q/1 -> Product/1  "psi_q_LUT"
  Gain2/1 -> Product1/2, Product/2
  psi_d/1 -> Product1/1  "psi_d_LUT"
  omega_m/1 -> Gain2/1
  i_d/1 -> Product2/1
  Ldq_LUT/1 -> Product2/2
  Sum6/1 -> u_q/1
  Product1/1 -> Sum6/2
  Product/1 -> Sum1/2
  Sum1/1 -> u_d/1
  i_q/1 -> Product3/1
  Lqd_LUT/1 -> Product3/2
  Product3/1 -> Sum6/1
  Product2/1 -> Sum1/1

== system gm_uz_pmsm_model_vnl/Curren t_Controller_With_FluxMaps_OLD/Entkopplungen/static_nonlinear_entkopplung ==
  psi_d : Inport
  psi_q : Inport  Port=2
  omega_m : Inport  Port=3
  Gain2 : Gain  Gain=polepair
  Product : Product  OutDataTypeStr=Inherit: Same as first input
  Product1 : Product
  Scope : Scope  NumInputPorts=2
  u_d : Outport
  u_q : Outport  Port=2
  wires:
  psi_q/1 -> Product/1  "psi_q_LUT"
  Gain2/1 -> Product1/2, Product/2
  Product1/1 -> Scope/1, u_q/1
  Product/1 -> Scope/2, u_d/1
  psi_d/1 -> Product1/1  "psi_d_LUT"
  omega_m/1 -> Gain2/1

== system gm_uz_pmsm_model_vnl/Curren t_Controller_With_FluxMaps_OLD/Psi_d_q/psid_approx ==
  Id : Inport
  Iq : Inport  Port=2
  FittingParameters : Inport  Port=3
  Demux : Demux  Outputs=23
  Log : Math  Operator=log  SignedPower=on
  Log1 : Math  Operator=log  SignedPower=on
  Product{,1..2,4..5,8} (6 alike) : Product  OutDataTypeStr=Inherit: Same as first input
  Product10 : Product  Inputs=3
  Product{3,6..7,12} (4 alike) : Product
  Sum : Sum  Inputs=|+-  OutDataTypeStr=Inherit: Same as first input
  Sum1 : Sum  Inputs=|+-
  Sum2 : Sum  Inputs=|+-  OutDataTypeStr=Inherit: Same as first input
  Sum3 : Sum  Inputs=|++-  OutDataTypeStr=Inherit: Same as first input
  Sum7 : Sum  Inputs=|+-  OutDataTypeStr=Inherit: Same as first input
  Tanh : Trigonometry  Operator=tanh
  Tanh1 : Trigonometry  Operator=tanh
  Tanh2 : Trigonometry  Operator=cosh
  Tanh3 : Trigonometry  Operator=cosh
  Terminator : Terminator
  psid : Outport
  wires:
  FittingParameters/1 -> Demux/1
  Demux/1 -> Product1/2  "ad1"
  Demux/3 -> Sum/2  "ad3"
  Sum/1 -> Product/1
  Demux/2 -> Product/2  "ad2"
  Product1/1 -> Sum7/1, Sum2/1  "psidself"
  Demux/4 -> Product3/2  "ad4"
  Sum1/1 -> Product2/1
  Demux/5 -> Product2/2  "ad5"
  Demux/6 -> Sum1/2  "ad6"
  Id/1 -> Sum1/1, Sum/1
  Product3/1 -> Sum2/2  "psid_s1"
  Iq/1 -> Product8/2, Product8/1, Product5/1, Product4/1
  Sum2/1 -> Product10/1  "psid_cross_s1"
  Tanh2/1 -> Log/1
  Tanh3/1 -> Log1/1
  Product8/1 -> Product7/1
  Product7/1 -> Sum3/2
  Demux/20 -> Product6/2
  Product6/1 -> Sum3/1
  Demux/19 -> Product12/2
  Product12/1 -> Sum3/3
  Sum3/1 -> Product10/2  "psiq_cross_s1_integrated"
  Demux/11 -> Product5/2  "aq5"
  Demux/8 -> Product4/2  "aq2"
  Product10/1 -> Sum7/2  "psid_cross"
  Sum7/1 -> psid/1  "psi_d_approx"
  Demux/14 -> Terminator/1
  Demux/13 -> Product10/3  "Reciprodical_F1G1"
  Log/1 -> Product6/1
  Log1/1 -> Product12/1
  Tanh/1 -> Product1/1
  Tanh1/1 -> Product3/1
  Product/1 -> Tanh/1
  Product2/1 -> Tanh1/1
  Product4/1 -> Tanh2/1
  Product5/1 -> Tanh3/1
  Demux/23 -> Product7/2

== system gm_uz_pmsm_model_vnl/Curren t_Controller_With_FluxMaps_OLD/Psi_d_q/psid_approx1 ==
  Id : Inport
  Iq : Inport  Port=2
  FittingParameters : Inport  Port=3
  Demux : Demux  Outputs=23
  Log : Math  Operator=log  SignedPower=on
  Log1 : Math  Operator=log  SignedPower=on
  Product{,1..2,4..5,8} (6 alike) : Product  OutDataTypeStr=Inherit: Same as first input
  Product10 : Product  Inputs=3
  Product{3,6..7,12} (4 alike) : Product
  Sum : Sum  Inputs=|+-  OutDataTypeStr=Inherit: Same as first input
  Sum1 : Sum  Inputs=|+-
  Sum2 : Sum  Inputs=|+-  OutDataTypeStr=Inherit: Same as first input
  Sum3 : Sum  Inputs=|++-  OutDataTypeStr=Inherit: Same as first input
  Sum7 : Sum  Inputs=|+-  OutDataTypeStr=Inherit: Same as first input
  Tanh : Trigonometry  Operator=tanh
  Tanh1 : Trigonometry  Operator=tanh
  Tanh2 : Trigonometry  Operator=cosh
  Tanh3 : Trigonometry  Operator=cosh
  Terminator : Terminator
  psid : Outport
  wires:
  FittingParameters/1 -> Demux/1
  Demux/1 -> Product1/2  "ad1"
  Demux/3 -> Sum/2  "ad3"
  Sum/1 -> Product/1
  Demux/2 -> Product/2  "ad2"
  Product1/1 -> Sum7/1, Sum2/1  "psidself"
  Demux/4 -> Product3/2  "ad4"
  Sum1/1 -> Product2/1
  Demux/5 -> Product2/2  "ad5"
  Demux/6 -> Sum1/2  "ad6"
  Id/1 -> Sum1/1, Sum/1
  Product3/1 -> Sum2/2  "psid_s1"
  Iq/1 -> Product8/2, Product8/1, Product5/1, Product4/1
  Sum2/1 -> Product10/1  "psid_cross_s1"
  Tanh2/1 -> Log/1
  Tanh3/1 -> Log1/1
  Product8/1 -> Product7/1
  Product7/1 -> Sum3/2
  Demux/20 -> Product6/2
  Product6/1 -> Sum3/1
  Demux/19 -> Product12/2
  Product12/1 -> Sum3/3
  Sum3/1 -> Product10/2  "psiq_cross_s1_integrated"
  Demux/11 -> Product5/2  "aq5"
  Demux/8 -> Product4/2  "aq2"
  Product10/1 -> Sum7/2  "psid_cross"
  Sum7/1 -> psid/1  "psi_d_approx"
  Demux/14 -> Terminator/1
  Demux/13 -> Product10/3  "Reciprodical_F1G1"
  Log/1 -> Product6/1
  Log1/1 -> Product12/1
  Tanh/1 -> Product1/1
  Tanh1/1 -> Product3/1
  Product/1 -> Tanh/1
  Product2/1 -> Tanh1/1
  Product4/1 -> Tanh2/1
  Product5/1 -> Tanh3/1
  Demux/23 -> Product7/2

== system gm_uz_pmsm_model_vnl/Curren t_Controller_With_FluxMaps_OLD/Psi_d_q/psiq_approx ==
  Id : Inport
  Iq : Inport  Port=2
  FittingParameters : Inport  Port=3
  Demux : Demux  Outputs=23
  Log1 : Math  Operator=log  SignedPower=on
  Log2 : Math  Operator=log  SignedPower=on
  Product{,2,7,10} (4 alike) : Product  OutDataTypeStr=Inherit: Same as first input
  Product{1,3..6,9} (6 alike) : Product
  Product20 : Product  Inputs=3
  Sum1 : Sum  Inputs=|++
  Sum10 : Sum  Inputs=|+-
  Sum2 : Sum  Inputs=|+-
  Sum3 : Sum  Inputs=-+|
  Sum4 : Sum  Inputs=++|
  Sum5 : Sum  Inputs=|+-
  Sum6 : Sum  Inputs=-+|
  Tanh : Trigonometry  Operator=tanh
  Tanh1 : Trigonometry  Operator=tanh
  Tanh2 : Trigonometry  Operator=cosh
  Tanh4 : Trigonometry  Operator=cosh
  psiq : Outport
  wires:
  FittingParameters/1 -> Demux/1
  Sum2/1 -> Product20/1  "psiq_cross_s1"
  Demux/10 -> Product3/2  "aq4"
  Demux/12 -> Product6/2  "aq6"
  Demux/8 -> Product/2  "aq2"
  Demux/11 -> Product2/2  "aq5"
  Demux/7 -> Product1/2  "aq1"
  Iq/1 -> Product2/1, Product6/1, Product/1, Product5/1
  Demux/9 -> Product5/2  "aq3"
  Tanh4/1 -> Log2/1
  Demux/22 -> Product4/1
  Product1/1 -> Sum4/2
  Product5/1 -> Sum4/1
  Sum4/1 -> Sum10/1, Sum2/1  "psiq_self"
  Sum1/1 -> Sum2/2
  Product3/1 -> Sum1/1  "psiq_s1"
  Product6/1 -> Sum1/2
  Sum3/1 -> Product7/2  "psid_cross_s1"
  Product7/1 -> Tanh4/1  "psid_s1"
  Product4/1 -> Sum5/1
  Product9/1 -> Sum5/2
  Product10/1 -> Tanh2/1  "psid_s1"
  Tanh2/1 -> Log1/1
  Demux/21 -> Product9/1
  Sum6/1 -> Product10/2  "psid_cross_s1"
  Demux/3 -> Sum3/1  "ad3"
  Demux/2 -> Product7/1  "ad2"
  Demux/5 -> Product10/1  "ad5"
  Demux/6 -> Sum6/1  "ad6"
  Id/1 -> Sum6/2, Sum3/2
  Sum5/1 -> Product20/2  "psid_cross_s1_integrated"
  Product20/1 -> Sum10/2  "psiq_cross"
  Sum10/1 -> psiq/1  "psiq_approx"
  Demux/14 -> Product20/3
  Log1/1 -> Product9/2
  Log2/1 -> Product4/2
  Tanh1/1 -> Product3/1
  Tanh/1 -> Product1/1
  Product2/1 -> Tanh1/1
  Product/1 -> Tanh/1

== system gm_uz_pmsm_model_vnl/Curren t_Controller_With_FluxMaps_OLD/Psi_d_q/psiq_approx1 ==
  Id : Inport
  Iq : Inport  Port=2
  FittingParameters : Inport  Port=3
  Demux : Demux  Outputs=23
  Log1 : Math  Operator=log  SignedPower=on
  Log2 : Math  Operator=log  SignedPower=on
  Product{,2,7,10} (4 alike) : Product  OutDataTypeStr=Inherit: Same as first input
  Product{1,3..6,9} (6 alike) : Product
  Product20 : Product  Inputs=3
  Sum1 : Sum  Inputs=|++
  Sum10 : Sum  Inputs=|+-  OutDataTypeStr=Inherit: Same as first input
  Sum2 : Sum  Inputs=|+-
  Sum3 : Sum  Inputs=-+|
  Sum4 : Sum  Inputs=++|
  Sum5 : Sum  Inputs=|+-
  Sum6 : Sum  Inputs=-+|
  Tanh : Trigonometry  Operator=tanh
  Tanh1 : Trigonometry  Operator=tanh
  Tanh2 : Trigonometry  Operator=cosh
  Tanh4 : Trigonometry  Operator=cosh
  psiq : Outport
  wires:
  FittingParameters/1 -> Demux/1
  Sum2/1 -> Product20/1  "psiq_cross_s1"
  Demux/10 -> Product3/2  "aq4"
  Demux/12 -> Product6/2  "aq6"
  Demux/8 -> Product/2  "aq2"
  Demux/11 -> Product2/2  "aq5"
  Demux/7 -> Product1/2  "aq1"
  Iq/1 -> Product2/1, Product6/1, Product/1, Product5/1
  Demux/9 -> Product5/2  "aq3"
  Tanh4/1 -> Log2/1
  Demux/22 -> Product4/1
  Product1/1 -> Sum4/2
  Product5/1 -> Sum4/1
  Sum4/1 -> Sum10/1, Sum2/1  "psiq_self"
  Sum1/1 -> Sum2/2
  Product3/1 -> Sum1/1  "psiq_s1"
  Product6/1 -> Sum1/2
  Sum3/1 -> Product7/2  "psid_cross_s1"
  Product7/1 -> Tanh4/1  "psid_s1"
  Product4/1 -> Sum5/1
  Product9/1 -> Sum5/2
  Product10/1 -> Tanh2/1  "psid_s1"
  Tanh2/1 -> Log1/1
  Demux/21 -> Product9/1
  Sum6/1 -> Product10/2  "psid_cross_s1"
  Demux/3 -> Sum3/1  "ad3"
  Demux/2 -> Product7/1  "ad2"
  Demux/5 -> Product10/1  "ad5"
  Demux/6 -> Sum6/1  "ad6"
  Id/1 -> Sum6/2, Sum3/2
  Sum5/1 -> Product20/2  "psid_cross_s1_integrated"
  Product20/1 -> Sum10/2  "psiq_cross"
  Sum10/1 -> psiq/1  "psiq_approx"
  Demux/14 -> Product20/3
  Log1/1 -> Product9/2
  Log2/1 -> Product4/2
  Tanh1/1 -> Product3/1
  Tanh/1 -> Product1/1
  Product2/1 -> Tanh1/1
  Product/1 -> Tanh/1

== system gm_uz_pmsm_model_vnl/Curren t_Controller_With_FluxMaps_OLD/Psi_d_q1/Ldd_approx1 ==
  psiq_cross_s1_integrated : Inport
  Id : Inport  Port=2
  FittingParameters : Inport  Port=3
  Demux : Demux  Outputs=23
  Product{,1..3} (4 alike) : Product  OutDataTypeStr=single
  Product10 : Product  Inputs=3  OutDataTypeStr=single
  Product14 : Product
  Product15 : Product
  Reciprocal : Product  Inputs=/  RndMeth=Zero  SaturateOnIntegerOverflow=on
  Reciprocal1 : Product  Inputs=/  RndMeth=Zero  SaturateOnIntegerOverflow=on
  Sum : Sum  Inputs=|+-  OutDataTypeStr=single
  Sum1 : Sum  Inputs=|+-  OutDataTypeStr=single
  Sum2 : Sum  Inputs=|+-
  Sum7 : Sum  Inputs=|+-
  Tanh1 : Trigonometry  Operator=cosh
  Tanh4 : Trigonometry  Operator=cosh
  Ldd : Outport
  wires:
  FittingParameters/1 -> Demux/1
  Demux/3 -> Sum/2  "ad3"
  Sum/1 -> Product/1
  Demux/2 -> Product/2  "ad2"
  Product1/1 -> Sum7/1, Sum2/1  "psidself_abgeleitet"
  Sum1/1 -> Product2/1
  Demux/5 -> Product2/2  "ad5"
  Demux/6 -> Sum1/2  "ad6"
  Id/1 -> Sum1/1, Sum/1
  Product3/1 -> Sum2/2  "psid_s1"
  Sum2/1 -> Product10/1  "psid_cross_s1_abgeleitet"
  Product10/1 -> Sum7/2  "psid_cross"
  Sum7/1 -> Ldd/1  "psid_cross_s1"
  Demux/13 -> Product10/3  "F1G1"
  Tanh4/1 -> Product14/1, Product14/2
  Tanh1/1 -> Product15/2, Product15/1
  Reciprocal1/1 -> Product3/1
  Product15/1 -> Reciprocal1/1
  Product14/1 -> Reciprocal/1
  Product/1 -> Tanh4/1
  Product2/1 -> Tanh1/1
  psiq_cross_s1_integrated/1 -> Product10/2
  Reciprocal/1 -> Product1/1
  Demux/15 -> Product3/2  "ad4*ad5"
  Demux/16 -> Product1/2  "ad1*ad2"

== system gm_uz_pmsm_model_vnl/Curren t_Controller_With_FluxMaps_OLD/Psi_d_q1/Lqq_approx1 ==
  psid_cross_s1_integrated : Inport
  Iq : Inport  Port=2
  FittingParameters : Inport  Port=3
  Demux : Demux  Outputs=23
  Product : Product  OutDataTypeStr=Inherit: Same as first input
  Product1 : Product
  Product14 : Product  OutDataTypeStr=Inherit: Same as first input
  Product15 : Product
  Product2 : Product  OutDataTypeStr=Inherit: Same as first input
  Product20 : Product  Inputs=3
  Product3 : Product
  Reciprocal : Product  Inputs=/  RndMeth=Zero  SaturateOnIntegerOverflow=on
  Reciprocal1 : Product  Inputs=/  RndMeth=Zero  SaturateOnIntegerOverflow=on
  Sum1 : Sum  Inputs=|++
  Sum10 : Sum  Inputs=|+-
  Sum2 : Sum  Inputs=|+-
  Sum4 : Sum  Inputs=|++
  Tanh1 : Trigonometry  Operator=cosh
  Tanh3 : Trigonometry  Operator=cosh
  Lqq : Outport
  wires:
  FittingParameters/1 -> Demux/1
  Demux/12 -> Sum4/2  "aq6"
  Product20/1 -> Sum10/2  "psiq_cross"
  Sum10/1 -> Lqq/1  "Lqq"
  Demux/14 -> Product20/3
  Demux/9 -> Sum1/2  "aq3"
  Tanh3/1 -> Product14/1, Product14/2
  Tanh1/1 -> Product15/2, Product15/1
  Sum2/1 -> Product20/1
  Reciprocal/1 -> Product1/1
  Reciprocal1/1 -> Product3/1
  Demux/8 -> Product/2  "aq2"
  Iq/1 -> Product2/1, Product/1
  Demux/11 -> Product2/2  "aq5"
  Product1/1 -> Sum1/1  "psidself_abgeleitet"
  Sum1/1 -> Sum10/1, Sum2/1
  Sum4/1 -> Sum2/2
  Product3/1 -> Sum4/1  "psid_s1"
  Product15/1 -> Reciprocal1/1
  Product2/1 -> Tanh1/1
  Product/1 -> Tanh3/1
  Product14/1 -> Reciprocal/1
  psid_cross_s1_integrated/1 -> Product20/2
  Demux/18 -> Product1/2  "aq1*aq2"
  Demux/17 -> Product3/2  "aq4*aq5"

== system gm_uz_pmsm_model_vnl/Curren t_Controller_With_FluxMaps_OLD/Psi_d_q1/psid_approx ==
  Id : Inport
  Iq : Inport  Port=2
  FittingParameters : Inport  Port=3
  Demux : Demux  Outputs=23
  Log : Math  Operator=log  SignedPower=on
  Log1 : Math  Operator=log  SignedPower=on
  Product{,1..2,4..5,8} (6 alike) : Product  OutDataTypeStr=Inherit: Same as first input
  Product10 : Product  Inputs=3
  Product{3,6..7,12} (4 alike) : Product
  Sum : Sum  Inputs=|+-  OutDataTypeStr=Inherit: Same as first input
  Sum1 : Sum  Inputs=|+-
  Sum2 : Sum  Inputs=|+-  OutDataTypeStr=Inherit: Same as first input
  Sum3 : Sum  Inputs=|++-  OutDataTypeStr=Inherit: Same as first input
  Sum7 : Sum  Inputs=|+-  OutDataTypeStr=Inherit: Same as first input
  Tanh : Trigonometry  Operator=tanh
  Tanh1 : Trigonometry  Operator=tanh
  Tanh2 : Trigonometry  Operator=cosh
  Tanh3 : Trigonometry  Operator=cosh
  Terminator : Terminator
  psid : Outport
  psiq_cross_s1_integrated : Outport  Port=2
  wires:
  FittingParameters/1 -> Demux/1
  Demux/1 -> Product1/2  "ad1"
  Demux/3 -> Sum/2  "ad3"
  Sum/1 -> Product/1
  Demux/2 -> Product/2  "ad2"
  Product1/1 -> Sum7/1, Sum2/1  "psidself"
  Demux/4 -> Product3/2  "ad4"
  Sum1/1 -> Product2/1
  Demux/5 -> Product2/2  "ad5"
  Demux/6 -> Sum1/2  "ad6"
  Id/1 -> Sum1/1, Sum/1
  Product3/1 -> Sum2/2  "psid_s1"
  Iq/1 -> Product8/2, Product8/1, Product5/1, Product4/1
  Sum2/1 -> Product10/1  "psid_cross_s1"
  Tanh2/1 -> Log/1
  Tanh3/1 -> Log1/1
  Product8/1 -> Product7/1
  Product7/1 -> Sum3/2
  Demux/20 -> Product6/2
  Product6/1 -> Sum3/1
  Demux/19 -> Product12/2
  Product12/1 -> Sum3/3
  Sum3/1 -> Product10/2, psiq_cross_s1_integrated/1  "psiq_cross_s1_integrated"
  Demux/11 -> Product5/2  "aq5"
  Demux/8 -> Product4/2  "aq2"
  Product10/1 -> Sum7/2  "psid_cross"
  Sum7/1 -> psid/1  "psi_d_approx"
  Demux/14 -> Terminator/1
  Demux/13 -> Product10/3  "Reciprodical_F1G1"
  Log/1 -> Product6/1
  Log1/1 -> Product12/1
  Tanh/1 -> Product1/1
  Tanh1/1 -> Product3/1
  Product/1 -> Tanh/1
  Product2/1 -> Tanh1/1
  Product4/1 -> Tanh2/1
  Product5/1 -> Tanh3/1
  Demux/23 -> Product7/2

== system gm_uz_pmsm_model_vnl/Curren t_Controller_With_FluxMaps_OLD/Psi_d_q1/psiq_approx ==
  Id : Inport
  Iq : Inport  Port=2
  FittingParameters : Inport  Port=3
  Demux : Demux  Outputs=23
  Log1 : Math  Operator=log  SignedPower=on
  Log2 : Math  Operator=log  SignedPower=on
  Product{,2,7,10} (4 alike) : Product  OutDataTypeStr=Inherit: Same as first input
  Product{1,3..6,9} (6 alike) : Product
  Product20 : Product  Inputs=3
  Sum1 : Sum  Inputs=|++
  Sum10 : Sum  Inputs=|+-
  Sum2 : Sum  Inputs=|+-
  Sum3 : Sum  Inputs=-+|
  Sum4 : Sum  Inputs=++|
  Sum5 : Sum  Inputs=|+-
  Sum6 : Sum  Inputs=-+|
  Tanh : Trigonometry  Operator=tanh
  Tanh1 : Trigonometry  Operator=tanh
  Tanh2 : Trigonometry  Operator=cosh
  Tanh4 : Trigonometry  Operator=cosh
  psiq : Outport
  psid_cross_s1_integrated : Outport  Port=2
  wires:
  FittingParameters/1 -> Demux/1
  Sum2/1 -> Product20/1  "psiq_cross_s1"
  Demux/10 -> Product3/2  "aq4"
  Demux/12 -> Product6/2  "aq6"
  Demux/8 -> Product/2  "aq2"
  Demux/11 -> Product2/2  "aq5"
  Demux/7 -> Product1/2  "aq1"
  Iq/1 -> Product2/1, Product6/1, Product/1, Product5/1
  Demux/9 -> Product5/2  "aq3"
  Tanh4/1 -> Log2/1
  Demux/22 -> Product4/1
  Product1/1 -> Sum4/2
  Product5/1 -> Sum4/1
  Sum4/1 -> Sum10/1, Sum2/1  "psiq_self"
  Sum1/1 -> Sum2/2
  Product3/1 -> Sum1/1  "psiq_s1"
  Product6/1 -> Sum1/2
  Sum3/1 -> Product7/2  "psid_cross_s1"
  Product7/1 -> Tanh4/1  "psid_s1"
  Product4/1 -> Sum5/1
  Product9/1 -> Sum5/2
  Product10/1 -> Tanh2/1  "psid_s1"
  Tanh2/1 -> Log1/1
  Demux/21 -> Product9/1
  Sum6/1 -> Product10/2  "psid_cross_s1"
  Demux/3 -> Sum3/1  "ad3"
  Demux/2 -> Product7/1  "ad2"
  Demux/5 -> Product10/1  "ad5"
  Demux/6 -> Sum6/1  "ad6"
  Id/1 -> Sum6/2, Sum3/2
  Sum5/1 -> psid_cross_s1_integrated/1, Product20/2  "psid_cross_s1_integrated"
  Product20/1 -> Sum10/2  "psiq_cross"
  Sum10/1 -> psiq/1  "psiq_approx"
  Demux/14 -> Product20/3
  Log1/1 -> Product9/2
  Log2/1 -> Product4/2
  Tanh1/1 -> Product3/1
  Tanh/1 -> Product1/1
  Product2/1 -> Tanh1/1
  Product/1 -> Tanh/1

== system gm_uz_pmsm_model_vnl/Curren t_Controller_With_FluxMaps_OLD/Psi_d_q2/Ldd_approx1 ==
  psiq_cross_s1_integrated : Inport
  Id : Inport  Port=2
  FittingParameters : Inport  Port=3
  Demux : Demux  Outputs=23
  Product{,1..3} (4 alike) : Product  OutDataTypeStr=single
  Product10 : Product  Inputs=3  OutDataTypeStr=single
  Product14 : Product
  Product15 : Product
  Reciprocal : Product  Inputs=/  RndMeth=Zero  SaturateOnIntegerOverflow=on
  Reciprocal1 : Product  Inputs=/  RndMeth=Zero  SaturateOnIntegerOverflow=on
  Sum : Sum  Inputs=|+-  OutDataTypeStr=single
  Sum1 : Sum  Inputs=|+-  OutDataTypeStr=single
  Sum2 : Sum  Inputs=|+-
  Sum7 : Sum  Inputs=|+-
  Tanh1 : Trigonometry  Operator=cosh
  Tanh4 : Trigonometry  Operator=cosh
  Ldd : Outport
  wires:
  FittingParameters/1 -> Demux/1
  Demux/3 -> Sum/2  "ad3"
  Sum/1 -> Product/1
  Demux/2 -> Product/2  "ad2"
  Product1/1 -> Sum7/1, Sum2/1  "psidself_abgeleitet"
  Sum1/1 -> Product2/1
  Demux/5 -> Product2/2  "ad5"
  Demux/6 -> Sum1/2  "ad6"
  Id/1 -> Sum1/1, Sum/1
  Product3/1 -> Sum2/2  "psid_s1"
  Sum2/1 -> Product10/1  "psid_cross_s1_abgeleitet"
  Product10/1 -> Sum7/2  "psid_cross"
  Sum7/1 -> Ldd/1  "psid_cross_s1"
  Demux/13 -> Product10/3  "F1G1"
  Tanh4/1 -> Product14/1, Product14/2
  Tanh1/1 -> Product15/2, Product15/1
  Reciprocal1/1 -> Product3/1
  Product15/1 -> Reciprocal1/1
  Product14/1 -> Reciprocal/1
  Product/1 -> Tanh4/1
  Product2/1 -> Tanh1/1
  psiq_cross_s1_integrated/1 -> Product10/2
  Reciprocal/1 -> Product1/1
  Demux/15 -> Product3/2  "ad4*ad5"
  Demux/16 -> Product1/2  "ad1*ad2"

== system gm_uz_pmsm_model_vnl/Curren t_Controller_With_FluxMaps_OLD/Psi_d_q2/Lqq_approx1 ==
  psid_cross_s1_integrated : Inport
  Iq : Inport  Port=2
  FittingParameters : Inport  Port=3
  Demux : Demux  Outputs=23
  Product : Product  OutDataTypeStr=Inherit: Same as first input
  Product1 : Product
  Product14 : Product  OutDataTypeStr=Inherit: Same as first input
  Product15 : Product
  Product2 : Product  OutDataTypeStr=Inherit: Same as first input
  Product20 : Product  Inputs=3
  Product3 : Product
  Reciprocal : Product  Inputs=/  RndMeth=Zero  SaturateOnIntegerOverflow=on
  Reciprocal1 : Product  Inputs=/  RndMeth=Zero  SaturateOnIntegerOverflow=on
  Sum1 : Sum  Inputs=|++
  Sum10 : Sum  Inputs=|+-
  Sum2 : Sum  Inputs=|+-
  Sum4 : Sum  Inputs=|++
  Tanh1 : Trigonometry  Operator=cosh
  Tanh3 : Trigonometry  Operator=cosh
  Lqq : Outport
  wires:
  FittingParameters/1 -> Demux/1
  Demux/12 -> Sum4/2  "aq6"
  Product20/1 -> Sum10/2  "psiq_cross"
  Sum10/1 -> Lqq/1  "Lqq"
  Demux/14 -> Product20/3
  Demux/9 -> Sum1/2  "aq3"
  Tanh3/1 -> Product14/1, Product14/2
  Tanh1/1 -> Product15/2, Product15/1
  Sum2/1 -> Product20/1
  Reciprocal/1 -> Product1/1
  Reciprocal1/1 -> Product3/1
  Demux/8 -> Product/2  "aq2"
  Iq/1 -> Product2/1, Product/1
  Demux/11 -> Product2/2  "aq5"
  Product1/1 -> Sum1/1  "psidself_abgeleitet"
  Sum1/1 -> Sum10/1, Sum2/1
  Sum4/1 -> Sum2/2
  Product3/1 -> Sum4/1  "psid_s1"
  Product15/1 -> Reciprocal1/1
  Product2/1 -> Tanh1/1
  Product/1 -> Tanh3/1
  Product14/1 -> Reciprocal/1
  psid_cross_s1_integrated/1 -> Product20/2
  Demux/18 -> Product1/2  "aq1*aq2"
  Demux/17 -> Product3/2  "aq4*aq5"

== system gm_uz_pmsm_model_vnl/Curren t_Controller_With_FluxMaps_OLD/Psi_d_q2/psid_approx ==
  Id : Inport
  Iq : Inport  Port=2
  FittingParameters : Inport  Port=3
  Demux : Demux  Outputs=23
  Log : Math  Operator=log  SignedPower=on
  Log1 : Math  Operator=log  SignedPower=on
  Product{,1..2,4..5,8} (6 alike) : Product  OutDataTypeStr=Inherit: Same as first input
  Product10 : Product  Inputs=3
  Product{3,6..7,12} (4 alike) : Product
  Sum : Sum  Inputs=|+-  OutDataTypeStr=Inherit: Same as first input
  Sum1 : Sum  Inputs=|+-
  Sum2 : Sum  Inputs=|+-  OutDataTypeStr=Inherit: Same as first input
  Sum3 : Sum  Inputs=|++-  OutDataTypeStr=Inherit: Same as first input
  Sum7 : Sum  Inputs=|+-  OutDataTypeStr=Inherit: Same as first input
  Tanh : Trigonometry  Operator=tanh
  Tanh1 : Trigonometry  Operator=tanh
  Tanh2 : Trigonometry  Operator=cosh
  Tanh3 : Trigonometry  Operator=cosh
  Terminator : Terminator
  psid : Outport
  psiq_cross_s1_integrated : Outport  Port=2
  wires:
  FittingParameters/1 -> Demux/1
  Demux/1 -> Product1/2  "ad1"
  Demux/3 -> Sum/2  "ad3"
  Sum/1 -> Product/1
  Demux/2 -> Product/2  "ad2"
  Product1/1 -> Sum7/1, Sum2/1  "psidself"
  Demux/4 -> Product3/2  "ad4"
  Sum1/1 -> Product2/1
  Demux/5 -> Product2/2  "ad5"
  Demux/6 -> Sum1/2  "ad6"
  Id/1 -> Sum1/1, Sum/1
  Product3/1 -> Sum2/2  "psid_s1"
  Iq/1 -> Product8/2, Product8/1, Product5/1, Product4/1
  Sum2/1 -> Product10/1  "psid_cross_s1"
  Tanh2/1 -> Log/1
  Tanh3/1 -> Log1/1
  Product8/1 -> Product7/1
  Product7/1 -> Sum3/2
  Demux/20 -> Product6/2
  Product6/1 -> Sum3/1
  Demux/19 -> Product12/2
  Product12/1 -> Sum3/3
  Sum3/1 -> Product10/2, psiq_cross_s1_integrated/1  "psiq_cross_s1_integrated"
  Demux/11 -> Product5/2  "aq5"
  Demux/8 -> Product4/2  "aq2"
  Product10/1 -> Sum7/2  "psid_cross"
  Sum7/1 -> psid/1  "psi_d_approx"
  Demux/14 -> Terminator/1
  Demux/13 -> Product10/3  "Reciprodical_F1G1"
  Log/1 -> Product6/1
  Log1/1 -> Product12/1
  Tanh/1 -> Product1/1
  Tanh1/1 -> Product3/1
  Product/1 -> Tanh/1
  Product2/1 -> Tanh1/1
  Product4/1 -> Tanh2/1
  Product5/1 -> Tanh3/1
  Demux/23 -> Product7/2
